simulink model "week2_problem3"  (R2019b)
settings: Solver=VariableStepAuto  StartTime=0.0  StopTime=120.0  RelTol=1e-3
model workspace (MAT data in the model file):
  b = 50
  m = 1000
  u = 500
settings Model: Creator=Shreyas  LastModifiedBy=Shreyas

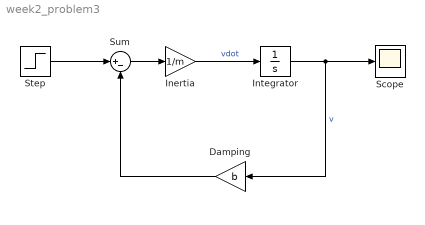
== system week2_problem3 ==
  Damping : Gain  Gain=b
  Inertia : Gain  Gain=1/m
  Integrator : Integrator
  Scope : Scope
  Step : Step  After=u  SampleTime=0
  Sum : Sum  Inputs=|+-
  wires:
  Integrator/1 -> Scope/1, Damping/1  "v"
  Inertia/1 -> Integrator/1  "vdot"
  Sum/1 -> Inertia/1
  Damping/1 -> Sum/2
  Step/1 -> Sum/1
